simulink model "chap2_3sim"  (R2015a)
settings: Solver=ode3  StartTime=0.0  StopTime=RunTime  FixedStep=0.01  RelTol=1e-3
settings Model: Creator=Masoud  LastModifiedBy=MSD
settings DebuggingCC: InheritedTsInSrcMsg=none  DiscreteInheritContinuousMsg=none

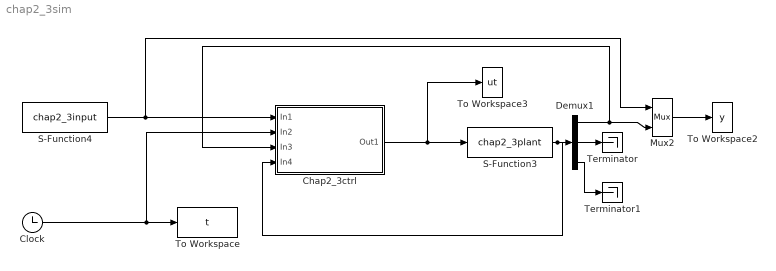
== system chap2_3sim ==
  Chap2_3ctrl : Subsystem
  Clock : Clock
  Demux1 : Demux  Outputs=3
  Mux2 : Mux  Inputs=2
  S-Function3 : S-Function  FunctionName=chap2_3plant  SFunctionModules='chap2_3plant'
  S-Function4 : S-Function  FunctionName=chap2_3input  SFunctionModules='chap2_3input'
  Terminator : Terminator
  Terminator1 : Terminator
  To Workspace : ToWorkspace  VariableName=t  SampleTime=-1
  To Workspace2 : ToWorkspace  VariableName=y  SampleTime=-1
  To Workspace3 : ToWorkspace  VariableName=ut  SampleTime=-1
  wires:
  Mux2/1 -> To Workspace2/1
  S-Function3/1 -> Chap2_3ctrl/4(In4), Demux1/1
  Demux1/2 -> Terminator/1
  Demux1/3 -> Terminator1/1
  Demux1/1 -> Chap2_3ctrl/3(In3), Mux2/2
  Chap2_3ctrl/1(Out1) -> To Workspace3/1, S-Function3/1
  Clock/1 -> Chap2_3ctrl/2(In2), To Workspace/1
  S-Function4/1 -> Mux2/1, Chap2_3ctrl/1(In1)

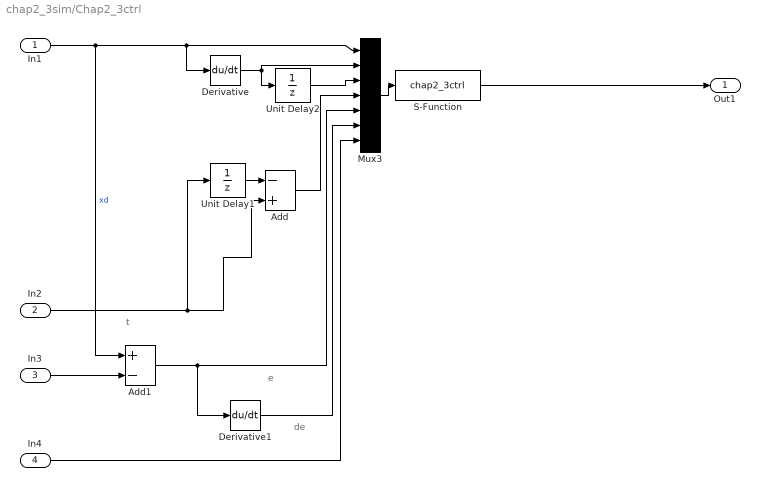
== system chap2_3sim/Chap2_3ctrl ==
  note: t
  note: de
  note: e
  In1 : Inport
  In2 : Inport  Port=2
  In3 : Inport  Port=3
  In4 : Inport  Port=4
  Add : Sum  Inputs=-+
  Add1 : Sum  Inputs=+-
  Derivative : Derivative
  Derivative1 : Derivative
  Mux3 : Mux  Inputs=7
  S-Function : S-Function  FunctionName=chap2_3ctrl  SFunctionModules='chap2_3ctrl'
  Unit Delay1 : UnitDelay  SampleTime=-1
  Unit Delay2 : UnitDelay  SampleTime=-1
  Out1 : Outport
  wires:
  S-Function/1 -> Out1/1
  In2/1 -> Add/2, Unit Delay1/1
  In4/1 -> Mux3/7
  Unit Delay2/1 -> Mux3/3
  Derivative/1 -> Mux3/2, Unit Delay2/1
  Mux3/1 -> S-Function/1
  Add/1 -> Mux3/4
  In1/1 -> Add1/1, Derivative/1, Mux3/1  "xd"
  Unit Delay1/1 -> Add/1
  Derivative1/1 -> Mux3/6
  In3/1 -> Add1/2
  Add1/1 -> Derivative1/1, Mux3/5
